simulink model "gm_sampleModel1401_2_sub"  (R2023a)
settings: Solver=VariableStepAuto  StartTime=0.0  StopTime=10.0  RelTol=1e-3
libraries: simulink x1
settings Model: Creator=user1  LastModifiedBy=user1
settings OptimizationCC: BlockReduction=off  ConditionallyExecuteInputs=off
settings DebuggingCC: InheritedTsInSrcMsg=none

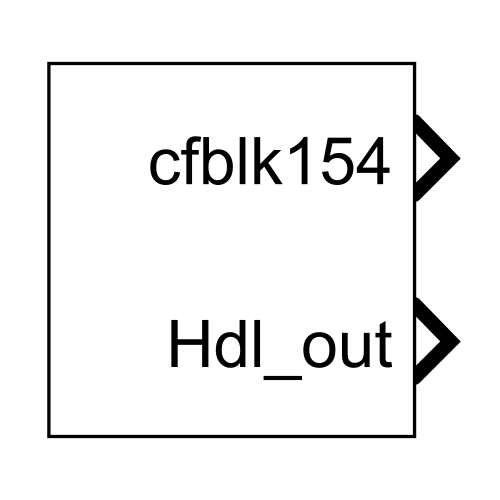
[thumbnail: Simulink's stored preview of the top-level diagram]
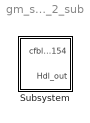
== system gm_sampleModel1401_2_sub ==
  Subsystem : Subsystem

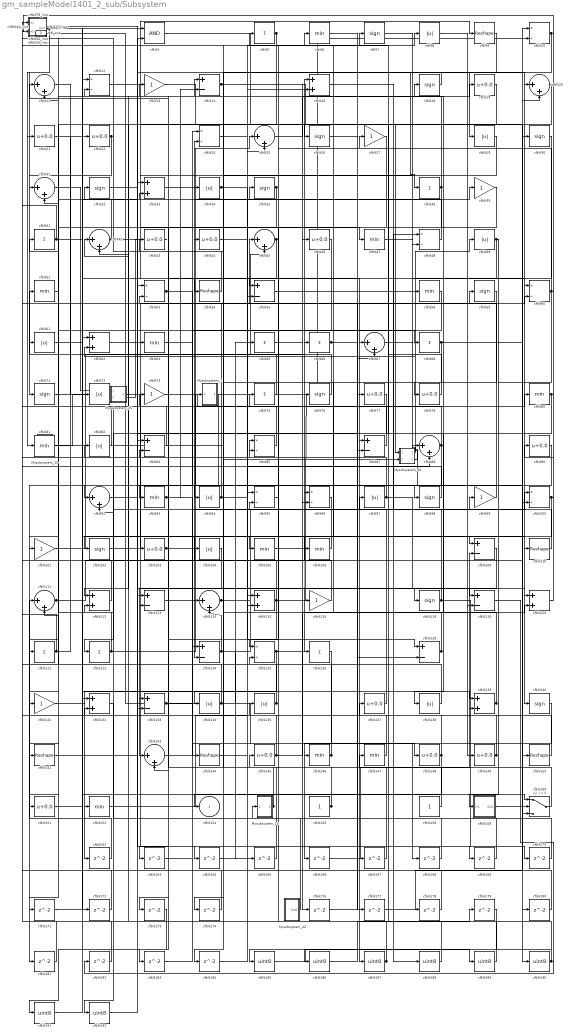
== system gm_sampleModel1401_2_sub/Subsystem ==
  Mysubsystem_10 : Subsystem
  Mysubsystem_19 : Subsystem
  Mysubsystem_25 : Subsystem
  Mysubsystem_40 : Subsystem
  Mysubsystem_42 : Subsystem
  Mysubsystem_7 : Subsystem
  cfblk{10,12,24,48,53,60,85,95..96,100,125} (11 alike) : Product  Inputs=*/  OutDataTypeStr=uint8  RndMeth=Zero  SaturateOnIntegerOverflow=on
  cfblk{13,27,39,73,99,101,116,131} (8 alike) : Gain  OutDataTypeStr=uint8
  cfblk{7,18,26,30,32,35,59,71,76,98,102,118,140} (13 alike) : Signum
  cfblk{19,21..22,43..44,46,77..78,90,103,137,145,148..149,151} (15 alike) : Bias  Bias=0.0  SaturateOnIntegerOverflow=off
  cfblk{8,29,34,49,61,72,82,94,97,104,134..135,138} (13 alike) : Abs  OutDataTypeStr=uint8  SaturateOnIntegerOverflow=off
  cfblk{6,47,51,58,63,80..81,93,105..106,146..147,152} (13 alike) : MinMax  OutDataTypeStr=uint8
  cfblk107_inst : Subsystem
  cfblk108_inst : Subsystem
  cfblk{14,55,83,87,109,113,119,124,128,133} (10 alike) : Sum  Inputs=+-  OutDataTypeStr=uint8
  cfblk{11,20,25,31,42,45,67,88,92,111,114,143} (12 alike) : Sum  Inputs=|++  OutDataTypeStr=uint8
  cfblk{9,54,110,141,144,150} (6 alike) : Reshape
  cfblk{16,33,62,112,115,120,132,139} (8 alike) : Sum  OutDataTypeStr=uint8
  cfblk{5,38,41,65..66,68,75,121..122,126} (10 alike) : Sum  Inputs=+  OutDataTypeStr=uint8
  cfblk127_inst : Subsystem
  cfblk129_inst : Subsystem
  cfblk136_inst : Subsystem
  cfblk142_inst : Subsystem
  cfblk156 : Constant  OutDataTypeStr=uint8  SampleTime=-1
  cfblk158 : Constant  OutDataTypeStr=uint8  SampleTime=-1
  cfblk159 : Subsystem
  cfblk15_inst : Subsystem
  cfblk160 : Switch  OutDataTypeStr=uint8  SaturateOnIntegerOverflow=off  InputSameDT=off
  cfblk{162..174,176..184} (22 alike) : Delay  SampleTime=1
  cfblk17_inst : Subsystem
  cfblk{185..192} (8 alike) : DataTypeConversion  OutDataTypeStr=uint8  SaturateOnIntegerOverflow=off  RndMeth=Floor
  cfblk2 : Constant  Value=0  OutDataTypeStr=uint8  SampleTime=1
  cfblk23_inst : Subsystem
  cfblk3 : Logic  AllPortsSameDT=off  OutDataTypeStr=boolean
  cfblk37_inst : Subsystem
  cfblk4 : Constant  Value=0  OutDataTypeStr=uint8  SampleTime=1
  cfblk40_inst : Subsystem
  cfblk50_inst : Subsystem
  cfblk56_inst : Subsystem
  cfblk79_inst : Subsystem
  cfblk154 : Outport  OutDataTypeStr=uint8  SampleTime=1  VectorParamsAs1DForOutWhenUnconnected=off
  Hdl_out : Outport  Port=2  OutDataTypeStr=uint8  SampleTime=1
  wires:
  Mysubsystem_10/1(Y) -> Mysubsystem_40/2(In2)
  Mysubsystem_19/1(Out1) -> cfblk145/1, cfblk53/2
  Mysubsystem_25/1(Out1) -> cfblk164/1
  Mysubsystem_40/1(Out1) -> cfblk49/1
  Mysubsystem_40/2(Out2) -> cfblk62/2
  Mysubsystem_42/1(Out1) -> Mysubsystem_19/1(In1)
  Mysubsystem_7/1(Out1) -> cfblk181/1
  cfblk10/1 -> cfblk29/1, cfblk140/1
  cfblk100/1 -> cfblk15_inst/2(in2), cfblk124/2
  cfblk101/1 -> cfblk45/2
  cfblk102/1 -> cfblk45/1
  cfblk103/1 -> cfblk25/1, cfblk95/2, cfblk80/1
  cfblk104/1 -> cfblk143/1
  cfblk105/1 -> cfblk100/1
  cfblk106/1 -> cfblk102/1
  cfblk107_inst/1(out1) -> cfblk71/1
  cfblk108_inst/1(out1) -> cfblk187/1
  cfblk109/1 -> cfblk113/2
  cfblk11/1 -> cfblk72/1
  cfblk110/1 -> cfblk40_inst/1(in1)
  cfblk111/1 -> cfblk30/1, cfblk16/1
  cfblk112/1 -> cfblk129_inst/1(in1)
  cfblk113/1 -> cfblk66/1
  cfblk114/1 -> cfblk134/1, cfblk58/1
  cfblk115/1 -> cfblk107_inst/2(in2), cfblk99/1, cfblk163/1
  cfblk116/1 -> cfblk24/2
  cfblk118/1 -> cfblk32/1, cfblk170/1
  cfblk119/1 -> cfblk182/1
  cfblk12/1 -> cfblk47/1
  cfblk120/1 -> cfblk90/1
  cfblk121/1 -> cfblk50_inst/2(in2), cfblk22/1
  cfblk122/1 -> cfblk142_inst/2(in2), cfblk39/1
  cfblk124/1 -> cfblk114/2, cfblk48/1, cfblk165/1
  cfblk125/1 -> cfblk76/1, cfblk162/1
  cfblk126/1 -> cfblk166/1
  cfblk127_inst/1(out1) -> cfblk26/1
  cfblk128/1 -> cfblk17_inst/2(in2), cfblk27/1
  cfblk129_inst/1(out1) -> cfblk37_inst/2(in2)
  cfblk13/1 -> cfblk46/1
  cfblk131/1 -> cfblk152/1
  cfblk132/1 -> cfblk191/1
  cfblk133/1 -> cfblk83/2, cfblk148/1
  cfblk134/1 -> cfblk42/2, cfblk168/1, Hdl_out/1, cfblk65/1
  cfblk135/1 -> cfblk35/1, cfblk33/2
  cfblk136_inst/1(out1) -> cfblk126/1
  cfblk137/1 -> cfblk79_inst/1(in1)
  cfblk138/1 -> cfblk40_inst/2(in2)
  cfblk139/1 -> cfblk18/1, cfblk6/1
  cfblk14/1 -> cfblk176/1, Mysubsystem_40/1(In1)
  cfblk140/1 -> cfblk146/1
  cfblk141/1 -> cfblk103/1
  cfblk142_inst/1(out1) -> cfblk48/2, cfblk177/1, cfblk63/1
  cfblk143/1 -> cfblk95/1
  cfblk144/1 -> cfblk25/2
  cfblk145/1 -> cfblk82/1, cfblk120/2
  cfblk146/1 -> cfblk135/1, cfblk111/2
  cfblk147/1 -> cfblk129_inst/2(in2)
  cfblk148/1 -> cfblk92/2, cfblk184/1
  cfblk149/1 -> cfblk137/1, cfblk109/2
  cfblk15_inst/1(out1) -> cfblk113/1
  cfblk150/1 -> cfblk132/2
  cfblk151/1 -> cfblk160/1
  cfblk152/1 -> cfblk115/1
  cfblk156/1 -> cfblk44/1, cfblk43/1
  cfblk158/1 -> cfblk147/1
  cfblk159/1(Out1) -> cfblk150/1
  cfblk16/1 -> cfblk188/1
  cfblk160/1 -> Mysubsystem_7/1(In1)
  cfblk162/1 -> cfblk111/1
  cfblk163/1 -> cfblk96/1
  cfblk164/1 -> cfblk88/2
  cfblk165/1 -> cfblk11/1
  cfblk166/1 -> cfblk139/2
  cfblk167/1 -> cfblk85/1
  cfblk168/1 -> cfblk112/2
  cfblk169/1 -> cfblk124/1
  cfblk17_inst/1(out1) -> cfblk9/1
  cfblk170/1 -> cfblk42/1
  cfblk171/1 -> cfblk62/1
  cfblk172/1 -> cfblk132/1
  cfblk173/1 -> cfblk192/1
  cfblk174/1 -> cfblk37_inst/1(in1)
  cfblk176/1 -> cfblk60/2
  cfblk177/1 -> cfblk10/1
  cfblk178/1 -> cfblk125/2
  cfblk179/1 -> cfblk185/1
  cfblk18/1 -> cfblk38/1
  cfblk180/1 -> cfblk107_inst/1(in1)
  cfblk181/1 -> cfblk23_inst/1(in1)
  cfblk182/1 -> cfblk79_inst/2(in2)
  cfblk183/1 -> cfblk24/1
  cfblk184/1 -> cfblk115/2
  cfblk185/1 -> cfblk189/1
  cfblk186/1 -> cfblk179/1
  cfblk187/1 -> cfblk85/2, cfblk12/2
  cfblk188/1 -> cfblk108_inst/1(in1)
  cfblk189/1 -> cfblk108_inst/2(in2)
  cfblk19/1 -> cfblk67/1
  cfblk190/1 -> cfblk97/1, cfblk186/1
  cfblk191/1 -> cfblk3/1
  cfblk192/1 -> cfblk3/2
  cfblk2/1 -> cfblk118/1
  cfblk20/1 -> cfblk112/1
  cfblk21/1 -> cfblk139/1
  cfblk22/1 -> cfblk31/2, cfblk31/1
  cfblk23_inst/1(out1) -> cfblk94/1
  cfblk24/1 -> cfblk7/1
  cfblk25/1 -> cfblk19/1
  cfblk26/1 -> cfblk67/2
  cfblk27/1 -> cfblk173/1
  cfblk29/1 -> cfblk154/1
  cfblk3/1 -> cfblk190/1
  cfblk30/1 -> cfblk93/1
  cfblk31/1 -> Mysubsystem_25/1(In1)
  cfblk32/1 -> cfblk169/1
  cfblk33/1 -> cfblk8/1
  cfblk34/1 -> cfblk14/1, cfblk128/1
  cfblk35/1 -> cfblk92/1, cfblk101/1
  cfblk37_inst/1(out1) -> cfblk81/1
  cfblk38/1 -> cfblk17_inst/1(in1), cfblk133/1, cfblk105/1
  cfblk39/1 -> cfblk151/1
  cfblk4/1 -> cfblk160/3
  cfblk40_inst/1(out1) -> cfblk20/1
  cfblk41/1 -> cfblk55/1, cfblk142_inst/1(in1)
  cfblk42/1 -> cfblk54/1, cfblk12/1
  cfblk43/1 -> Mysubsystem_25/2(In2)
  cfblk44/1 -> cfblk16/2
  cfblk45/1 -> cfblk55/2, cfblk5/1
  cfblk46/1 -> cfblk171/1
  cfblk47/1 -> cfblk60/1
  cfblk48/1 -> cfblk136_inst/2(in2)
  cfblk49/1 -> cfblk87/1, cfblk109/1
  cfblk5/1 -> cfblk141/1, cfblk127_inst/2(in2)
  cfblk50_inst/1(out1) -> cfblk21/1, cfblk119/1
  cfblk51/1 -> cfblk131/1
  cfblk53/1 -> cfblk100/2, cfblk68/1
  cfblk54/1 -> cfblk136_inst/1(in1)
  cfblk55/1 -> cfblk178/1
  cfblk56_inst/1(out1) -> cfblk83/1, cfblk172/1
  cfblk58/1 -> cfblk183/1
  cfblk59/1 -> cfblk78/1
  cfblk6/1 -> cfblk128/2
  cfblk60/1 -> cfblk23_inst/2(in2), cfblk159/1(In1)
  cfblk61/1 -> cfblk110/1
  cfblk62/1 -> cfblk116/1
  cfblk63/1 -> cfblk34/1
  cfblk65/1 -> cfblk167/1
  cfblk66/1 -> cfblk77/1, cfblk160/2, cfblk119/2
  cfblk67/1 -> cfblk180/1
  cfblk68/1 -> cfblk20/2, cfblk114/1, cfblk106/1
  cfblk7/1 -> cfblk88/1
  cfblk71/1 -> cfblk33/1
  cfblk72/1 -> cfblk10/2, Mysubsystem_10/1(In1)
  cfblk73/1 -> cfblk96/2
  cfblk75/1 -> cfblk13/1
  cfblk76/1 -> cfblk51/1
  cfblk77/1 -> cfblk143/2
  cfblk78/1 -> cfblk15_inst/1(in1)
  cfblk79_inst/1(out1) -> cfblk87/2
  cfblk8/1 -> cfblk149/1
  cfblk80/1 -> cfblk138/1, cfblk122/1
  cfblk81/1 -> cfblk121/1
  cfblk82/1 -> cfblk50_inst/1(in1)
  cfblk83/1 -> cfblk41/1
  cfblk85/1 -> cfblk73/1
  cfblk87/1 -> cfblk61/1
  cfblk88/1 -> cfblk133/2, cfblk11/2
  cfblk9/1 -> cfblk174/1
  cfblk90/1 -> cfblk104/1
  cfblk92/1 -> cfblk98/1
  cfblk93/1 -> cfblk144/1, cfblk14/2
  cfblk94/1 -> cfblk59/1, cfblk127_inst/1(in1)
  cfblk95/1 -> cfblk75/1
  cfblk96/1 -> cfblk125/1
  cfblk97/1 -> cfblk56_inst/1(in1), cfblk120/1
  cfblk98/1 -> cfblk56_inst/2(in2)
  cfblk99/1 -> cfblk53/1

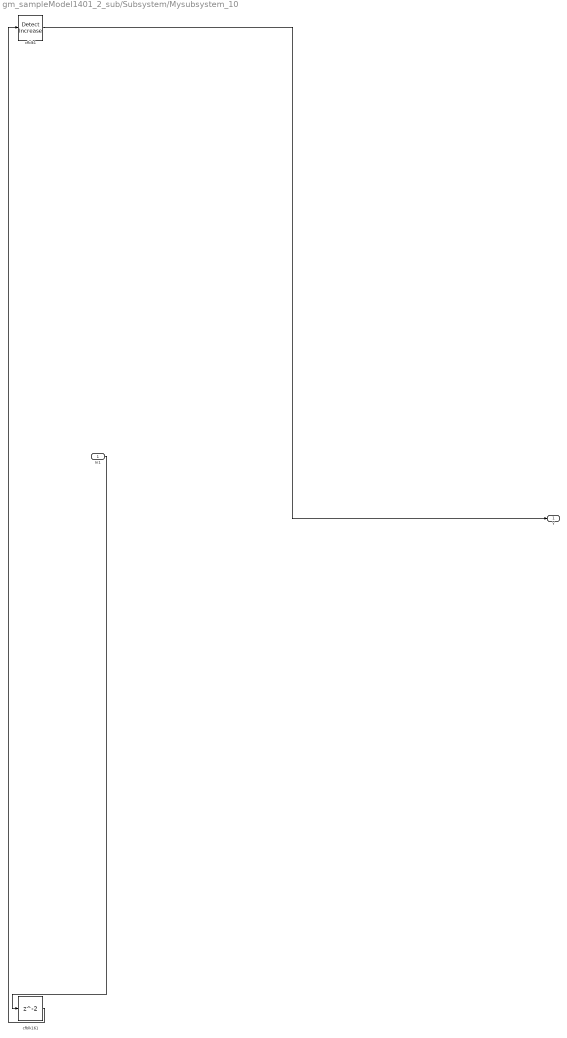
== system gm_sampleModel1401_2_sub/Subsystem/Mysubsystem_10 ==
  In1 : Inport  OutDataTypeStr=uint8  PortDimensions=1  SampleTime=1
  cfblk1 : simulink/Logic and Bit Operations/Detect Increase  vinit=0.0  OutDataTypeStr=boolean
      settings: LibrarySourceBlock=|
      | hdlsllib/Logic and Bit
      | Operations/Detect
      | Increase
  cfblk161 : Delay  SampleTime=1
  Y : Outport  SampleTime=1
  wires:
  In1/1 -> cfblk161/1
  cfblk1/1 -> Y/1
  cfblk161/1 -> cfblk1/1

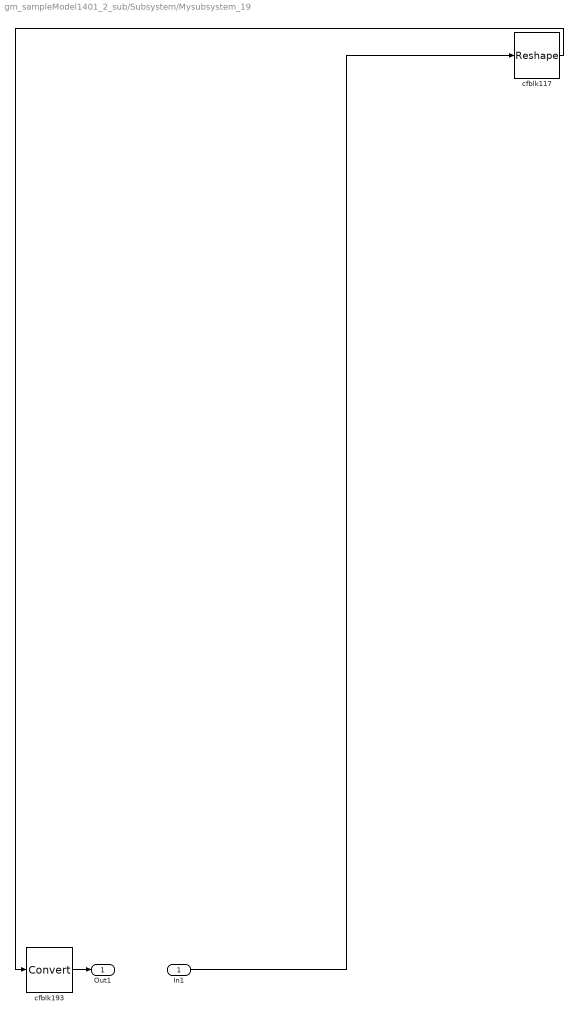
== system gm_sampleModel1401_2_sub/Subsystem/Mysubsystem_19 ==
  In1 : Inport  OutDataTypeStr=uint8  PortDimensions=1  SampleTime=1
  cfblk117 : Reshape
  cfblk193 : DataTypeConversion  SaturateOnIntegerOverflow=off  RndMeth=Floor
  Out1 : Outport  SampleTime=1
  wires:
  In1/1 -> cfblk117/1
  cfblk117/1 -> cfblk193/1
  cfblk193/1 -> Out1/1

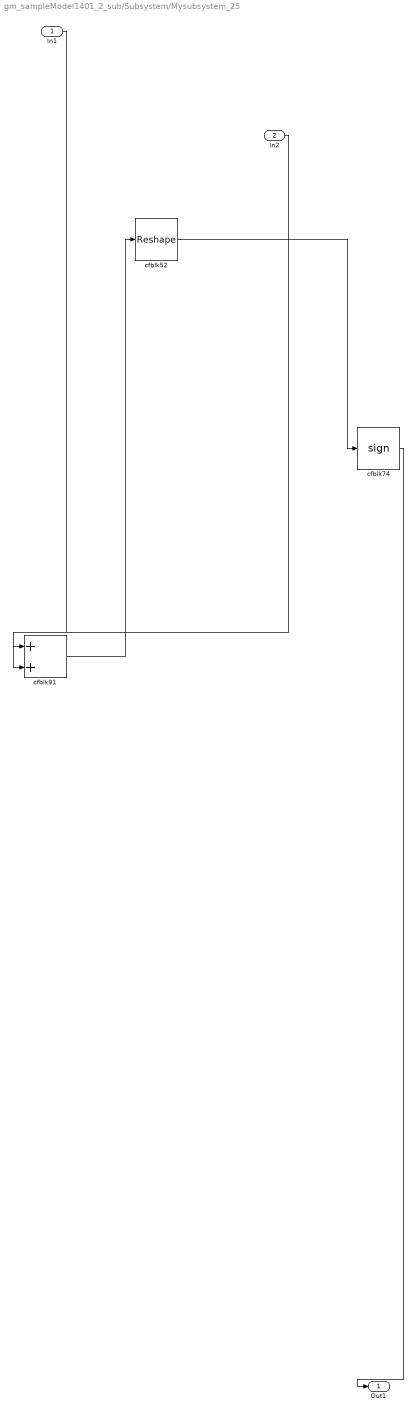
== system gm_sampleModel1401_2_sub/Subsystem/Mysubsystem_25 ==
  In1 : Inport  OutDataTypeStr=uint8  PortDimensions=1  SampleTime=1
  In2 : Inport  Port=2  OutDataTypeStr=uint8  PortDimensions=1  SampleTime=1
  cfblk52 : Reshape
  cfblk74 : Signum
  cfblk91 : Sum
  Out1 : Outport  SampleTime=1
  wires:
  In1/1 -> cfblk91/2
  In2/1 -> cfblk91/1
  cfblk52/1 -> cfblk74/1
  cfblk74/1 -> Out1/1
  cfblk91/1 -> cfblk52/1

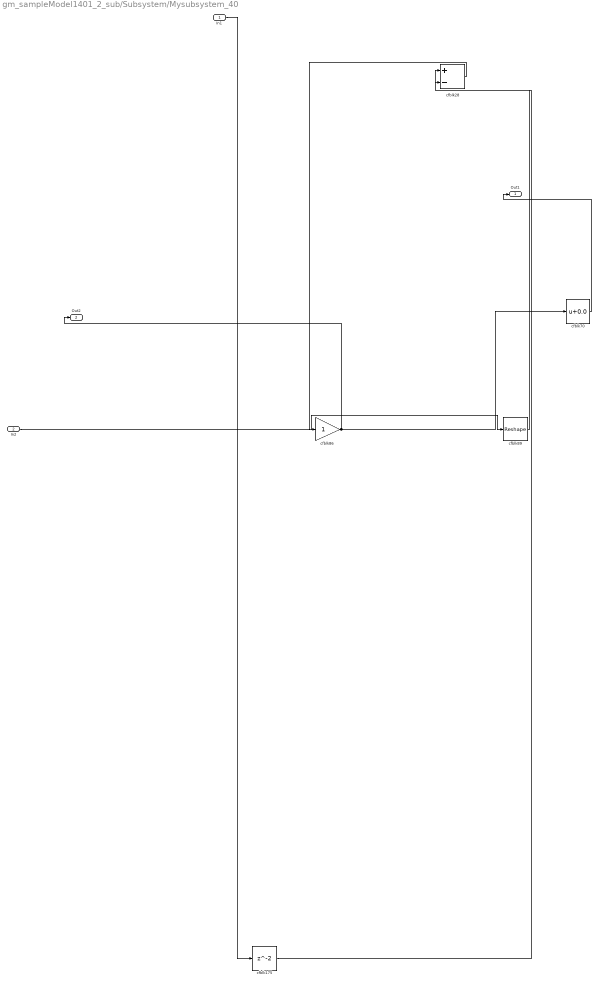
== system gm_sampleModel1401_2_sub/Subsystem/Mysubsystem_40 ==
  In1 : Inport  OutDataTypeStr=uint8  PortDimensions=1  SampleTime=1
  In2 : Inport  Port=2  OutDataTypeStr=boolean  PortDimensions=1  SampleTime=1
  cfblk175 : Delay  SampleTime=1
  cfblk28 : Sum  Inputs=+-
  cfblk70 : Bias  Bias=0.0  SaturateOnIntegerOverflow=off
  cfblk86 : Gain
  cfblk89 : Reshape
  Out1 : Outport  SampleTime=1
  Out2 : Outport  Port=2  SampleTime=1
  wires:
  In1/1 -> cfblk175/1
  In2/1 -> cfblk89/1
  cfblk175/1 -> cfblk28/1
  cfblk28/1 -> cfblk86/1
  cfblk70/1 -> Out1/1
  cfblk86/1 -> cfblk70/1, Out2/1
  cfblk89/1 -> cfblk28/2

== system gm_sampleModel1401_2_sub/Subsystem/Mysubsystem_42 ==
  cfblk157 : Subsystem  mask(Counter Limited){uplimit=double(7), tsamp=double(-1)}
      mask prompts: uplimit "Simulink:masks:UpperLimit_MP"; tsamp "Simulink:masks:SampleTime_MP"
      mask help: Simulink:masks:CounterLimited_MD
      mask init:
      | nbits = double(8);
      | tsamp = double(-1);
      | uplimit = double(7);
  cfblk194 : DataTypeConversion  OutDataTypeStr=uint8  SaturateOnIntegerOverflow=off  RndMeth=Floor
  Out1 : Outport  SampleTime=1
  wires:
  cfblk157/1(y) -> cfblk194/1
  cfblk194/1 -> Out1/1

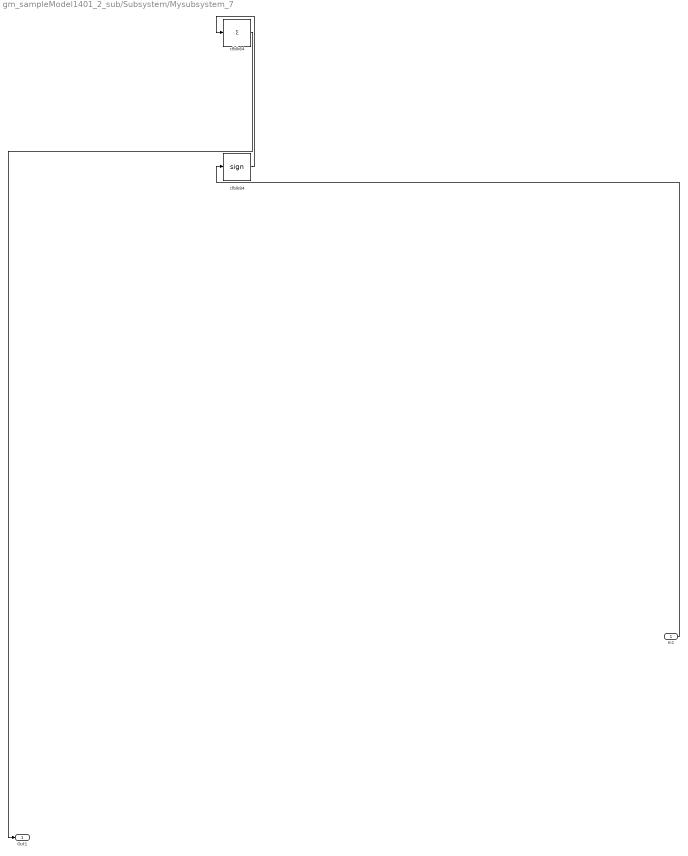
== system gm_sampleModel1401_2_sub/Subsystem/Mysubsystem_7 ==
  In1 : Inport  OutDataTypeStr=uint8  PortDimensions=1  SampleTime=1
  cfblk64 : Sum  Inputs=+
  cfblk84 : Signum
  Out1 : Outport  SampleTime=1
  wires:
  In1/1 -> cfblk84/1
  cfblk64/1 -> Out1/1
  cfblk84/1 -> cfblk64/1

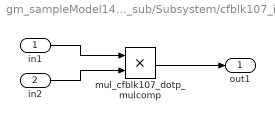
== system gm_sampleModel1401_2_sub/Subsystem/cfblk107_inst ==
  in1 : Inport  OutDataTypeStr=uint8  SampleTime=1
  in2 : Inport  Port=2  OutDataTypeStr=uint8  SampleTime=1
  mul_cfblk107_dotp_mulcomp : Product  Inputs=**  OutDataTypeStr=uint8  SampleTime=1
  out1 : Outport  OutDataTypeStr=uint8  SampleTime=1
  wires:
  in1/1 -> mul_cfblk107_dotp_mulcomp/1
  in2/1 -> mul_cfblk107_dotp_mulcomp/2
  mul_cfblk107_dotp_mulcomp/1 -> out1/1

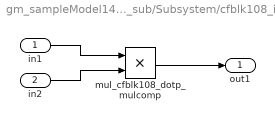
== system gm_sampleModel1401_2_sub/Subsystem/cfblk108_inst ==
  in1 : Inport  OutDataTypeStr=uint8  SampleTime=1
  in2 : Inport  Port=2  OutDataTypeStr=uint8  SampleTime=1
  mul_cfblk108_dotp_mulcomp : Product  Inputs=**  OutDataTypeStr=uint8  SampleTime=1
  out1 : Outport  OutDataTypeStr=uint8  SampleTime=1
  wires:
  in1/1 -> mul_cfblk108_dotp_mulcomp/1
  in2/1 -> mul_cfblk108_dotp_mulcomp/2
  mul_cfblk108_dotp_mulcomp/1 -> out1/1

== system gm_sampleModel1401_2_sub/Subsystem/cfblk127_inst ==
  in1 : Inport  OutDataTypeStr=uint8  SampleTime=1
  in2 : Inport  Port=2  OutDataTypeStr=uint8  SampleTime=1
  mul_cfblk127_dotp_mulcomp : Product  Inputs=**  OutDataTypeStr=uint8  SampleTime=1
  out1 : Outport  OutDataTypeStr=uint8  SampleTime=1
  wires:
  in1/1 -> mul_cfblk127_dotp_mulcomp/1
  in2/1 -> mul_cfblk127_dotp_mulcomp/2
  mul_cfblk127_dotp_mulcomp/1 -> out1/1

== system gm_sampleModel1401_2_sub/Subsystem/cfblk129_inst ==
  in1 : Inport  OutDataTypeStr=uint8  SampleTime=1
  in2 : Inport  Port=2  OutDataTypeStr=uint8  SampleTime=1
  mul_cfblk129_dotp_mulcomp : Product  Inputs=**  OutDataTypeStr=uint8  SampleTime=1
  out1 : Outport  OutDataTypeStr=uint8  SampleTime=1
  wires:
  in1/1 -> mul_cfblk129_dotp_mulcomp/1
  in2/1 -> mul_cfblk129_dotp_mulcomp/2
  mul_cfblk129_dotp_mulcomp/1 -> out1/1

== system gm_sampleModel1401_2_sub/Subsystem/cfblk136_inst ==
  in1 : Inport  OutDataTypeStr=uint8  SampleTime=1
  in2 : Inport  Port=2  OutDataTypeStr=uint8  SampleTime=1
  mul_cfblk136_dotp_mulcomp : Product  Inputs=**  OutDataTypeStr=uint8  SampleTime=1
  out1 : Outport  OutDataTypeStr=uint8  SampleTime=1
  wires:
  in1/1 -> mul_cfblk136_dotp_mulcomp/1
  in2/1 -> mul_cfblk136_dotp_mulcomp/2
  mul_cfblk136_dotp_mulcomp/1 -> out1/1

== system gm_sampleModel1401_2_sub/Subsystem/cfblk142_inst ==
  in1 : Inport  OutDataTypeStr=uint8  SampleTime=1
  in2 : Inport  Port=2  OutDataTypeStr=uint8  SampleTime=1
  mul_cfblk142_dotp_mulcomp : Product  Inputs=**  OutDataTypeStr=uint8  SampleTime=1
  out1 : Outport  OutDataTypeStr=uint8  SampleTime=1
  wires:
  in1/1 -> mul_cfblk142_dotp_mulcomp/1
  in2/1 -> mul_cfblk142_dotp_mulcomp/2
  mul_cfblk142_dotp_mulcomp/1 -> out1/1

== system gm_sampleModel1401_2_sub/Subsystem/cfblk159 ==
  In1 : Inport  OutDataTypeStr=uint8  PortDimensions=1  SampleTime=1
  Out1 : Outport  SampleTime=1
  wires:
  In1/1 -> Out1/1

== system gm_sampleModel1401_2_sub/Subsystem/cfblk15_inst ==
  in1 : Inport  OutDataTypeStr=uint8  SampleTime=1
  in2 : Inport  Port=2  OutDataTypeStr=uint8  SampleTime=1
  mul_cfblk15_dotp_mulcomp : Product  Inputs=**  OutDataTypeStr=uint8  SampleTime=1
  out1 : Outport  OutDataTypeStr=uint8  SampleTime=1
  wires:
  in1/1 -> mul_cfblk15_dotp_mulcomp/1
  in2/1 -> mul_cfblk15_dotp_mulcomp/2
  mul_cfblk15_dotp_mulcomp/1 -> out1/1

== system gm_sampleModel1401_2_sub/Subsystem/cfblk17_inst ==
  in1 : Inport  OutDataTypeStr=uint8  SampleTime=1
  in2 : Inport  Port=2  OutDataTypeStr=uint8  SampleTime=1
  mul_cfblk17_dotp_mulcomp : Product  Inputs=**  OutDataTypeStr=uint8  SampleTime=1
  out1 : Outport  OutDataTypeStr=uint8  SampleTime=1
  wires:
  in1/1 -> mul_cfblk17_dotp_mulcomp/1
  in2/1 -> mul_cfblk17_dotp_mulcomp/2
  mul_cfblk17_dotp_mulcomp/1 -> out1/1

== system gm_sampleModel1401_2_sub/Subsystem/cfblk23_inst ==
  in1 : Inport  OutDataTypeStr=uint8  SampleTime=1
  in2 : Inport  Port=2  OutDataTypeStr=uint8  SampleTime=1
  mul_cfblk23_dotp_mulcomp : Product  Inputs=**  OutDataTypeStr=uint8  SampleTime=1
  out1 : Outport  OutDataTypeStr=uint8  SampleTime=1
  wires:
  in1/1 -> mul_cfblk23_dotp_mulcomp/1
  in2/1 -> mul_cfblk23_dotp_mulcomp/2
  mul_cfblk23_dotp_mulcomp/1 -> out1/1

== system gm_sampleModel1401_2_sub/Subsystem/cfblk37_inst ==
  in1 : Inport  OutDataTypeStr=uint8  SampleTime=1
  in2 : Inport  Port=2  OutDataTypeStr=uint8  SampleTime=1
  mul_cfblk37_dotp_mulcomp : Product  Inputs=**  OutDataTypeStr=uint8  SampleTime=1
  out1 : Outport  OutDataTypeStr=uint8  SampleTime=1
  wires:
  in1/1 -> mul_cfblk37_dotp_mulcomp/1
  in2/1 -> mul_cfblk37_dotp_mulcomp/2
  mul_cfblk37_dotp_mulcomp/1 -> out1/1

== system gm_sampleModel1401_2_sub/Subsystem/cfblk40_inst ==
  in1 : Inport  OutDataTypeStr=uint8  SampleTime=1
  in2 : Inport  Port=2  OutDataTypeStr=uint8  SampleTime=1
  mul_cfblk40_dotp_mulcomp : Product  Inputs=**  OutDataTypeStr=uint8  SampleTime=1
  out1 : Outport  OutDataTypeStr=uint8  SampleTime=1
  wires:
  in1/1 -> mul_cfblk40_dotp_mulcomp/1
  in2/1 -> mul_cfblk40_dotp_mulcomp/2
  mul_cfblk40_dotp_mulcomp/1 -> out1/1

== system gm_sampleModel1401_2_sub/Subsystem/cfblk50_inst ==
  in1 : Inport  OutDataTypeStr=uint8  SampleTime=1
  in2 : Inport  Port=2  OutDataTypeStr=uint8  SampleTime=1
  mul_cfblk50_dotp_mulcomp : Product  Inputs=**  OutDataTypeStr=uint8  SampleTime=1
  out1 : Outport  OutDataTypeStr=uint8  SampleTime=1
  wires:
  in1/1 -> mul_cfblk50_dotp_mulcomp/1
  in2/1 -> mul_cfblk50_dotp_mulcomp/2
  mul_cfblk50_dotp_mulcomp/1 -> out1/1

== system gm_sampleModel1401_2_sub/Subsystem/cfblk56_inst ==
  in1 : Inport  OutDataTypeStr=uint8  SampleTime=1
  in2 : Inport  Port=2  OutDataTypeStr=uint8  SampleTime=1
  mul_cfblk56_dotp_mulcomp : Product  Inputs=**  OutDataTypeStr=uint8  SampleTime=1
  out1 : Outport  OutDataTypeStr=uint8  SampleTime=1
  wires:
  in1/1 -> mul_cfblk56_dotp_mulcomp/1
  in2/1 -> mul_cfblk56_dotp_mulcomp/2
  mul_cfblk56_dotp_mulcomp/1 -> out1/1

== system gm_sampleModel1401_2_sub/Subsystem/cfblk79_inst ==
  in1 : Inport  OutDataTypeStr=uint8  SampleTime=1
  in2 : Inport  Port=2  OutDataTypeStr=uint8  SampleTime=1
  mul_cfblk79_dotp_mulcomp : Product  Inputs=**  OutDataTypeStr=uint8  SampleTime=1
  out1 : Outport  OutDataTypeStr=uint8  SampleTime=1
  wires:
  in1/1 -> mul_cfblk79_dotp_mulcomp/1
  in2/1 -> mul_cfblk79_dotp_mulcomp/2
  mul_cfblk79_dotp_mulcomp/1 -> out1/1

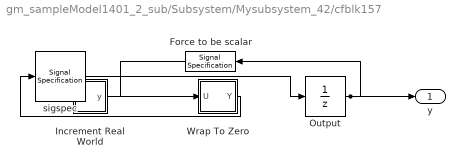
== system gm_sampleModel1401_2_sub/Subsystem/Mysubsystem_42/cfblk157 ==
  Force to be scalar : SignalSpecification  DisableCoverage=on  Dimensions=1
  Increment Real World : Subsystem  mask(Real World Value Increment){}
      mask help: Simulink:masks:RealWorldValueIncrement_MD
      mask Display: disp('V++')
  Output : UnitDelay  InitialCondition=0.0  SampleTime=tsamp  HasFrameUpgradeWarning=on
  Wrap To Zero : Subsystem  mask(Wrap To Zero){Threshold=double(7)}
      mask prompts: Threshold "Simulink:masks:Threshold_MP"
      mask help: Simulink:masks:WrapToZero_MD
  sigspec : SignalSpecification  OutDataTypeStr=uint8  Dimensions=1
  y : Outport  SampleTime=1
  wires:
  Force to be scalar/1 -> Increment Real World/1(u)
  Increment Real World/1(y) -> Wrap To Zero/1(U)
  Output/1 -> Force to be scalar/1, y/1
  Wrap To Zero/1(Y) -> sigspec/1
  sigspec/1 -> Output/1

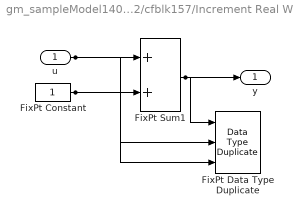
== system gm_sampleModel1401_2_sub/Subsystem/Mysubsystem_42/cfblk157/Increment Real World ==
  u : Inport  OutDataTypeStr=uint8  SampleTime=1
  FixPt Constant : Constant  DisableCoverage=on  OutDataTypeStr=Inherit: Inherit via back propagation  SampleTime=-1
  FixPt Data Type Duplicate : DataTypeDuplicate  DisableCoverage=on  NumInputPorts=3
  FixPt Sum1 : Sum  InputSameDT=on  OutDataTypeStr=Inherit: Inherit via back propagation  LockScale=on
  y : Outport  SampleTime=1
  wires:
  u/1 -> FixPt Sum1/1, FixPt Data Type Duplicate/2
  FixPt Constant/1 -> FixPt Sum1/2, FixPt Data Type Duplicate/3
  FixPt Sum1/1 -> FixPt Data Type Duplicate/1, y/1

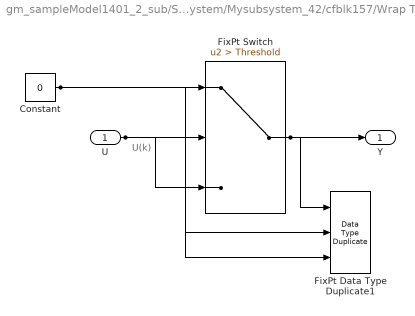
== system gm_sampleModel1401_2_sub/Subsystem/Mysubsystem_42/cfblk157/Wrap To Zero ==
  note: U(k)
  U : Inport  OutDataTypeStr=uint8  SampleTime=1
  Constant : Constant  DisableCoverage=on  Value=0  OutDataTypeStr=Inherit: Inherit via back propagation  SampleTime=-1
  FixPt Data Type Duplicate1 : DataTypeDuplicate  DisableCoverage=on  NumInputPorts=3
  FixPt Switch : Switch  Criteria=u2 > Threshold  Threshold=Threshold  OutDataTypeStr=Inherit: Inherit via back propagation  ZeroCross=off  SaturateOnIntegerOverflow=off  InputSameDT=off
  Y : Outport  SampleTime=1
  wires:
  U/1 -> FixPt Switch/3, FixPt Switch/2, FixPt Data Type Duplicate1/2
  Constant/1 -> FixPt Switch/1, FixPt Data Type Duplicate1/3
  FixPt Switch/1 -> FixPt Data Type Duplicate1/1, Y/1
